simulink model "test_hysteresis_sim"  (R2024a)
settings: Solver=VariableStepAuto  StartTime=0.0  StopTime=10.0  RelTol=1e-3
settings Model: Creator=pichim  LastModifiedBy=pichim

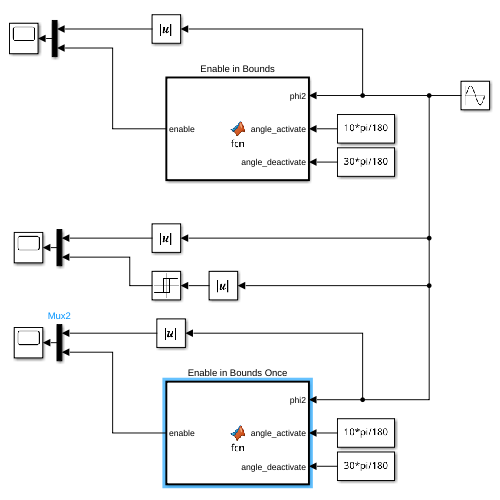
[thumbnail: Simulink's stored preview of the top-level diagram]
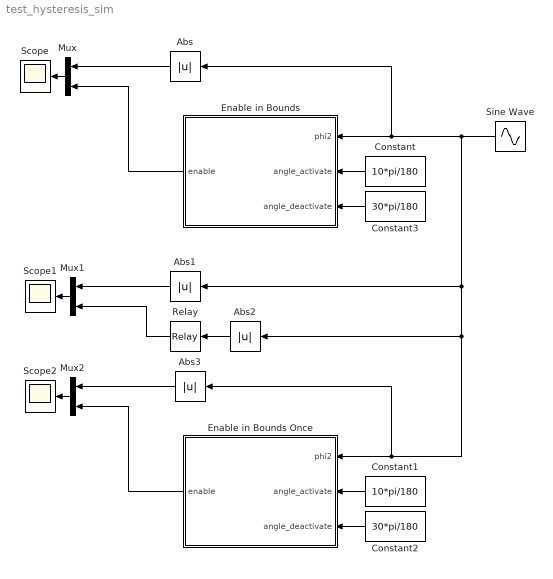
== system test_hysteresis_sim ==
  Abs{,1..3} (4 alike) : Abs  SaturateOnIntegerOverflow=off
  Constant : Constant  Value=10*pi/180
  Constant1 : Constant  Value=10*pi/180
  Constant2 : Constant  Value=30*pi/180
  Constant3 : Constant  Value=30*pi/180
  Enable in Bounds : MATLAB Function  TreatAsAtomicUnit=on
  Enable in Bounds Once : MATLAB Function  TreatAsAtomicUnit=on
  Mux : Mux  Inputs=2
  Mux1 : Mux  Inputs=2
  Mux2 : Mux  Inputs=2
  Relay : Relay  OnSwitchValue=30*pi/180  OffSwitchValue=10*pi/180  OnOutputValue=0  OffOutputValue=1
  Scope : Scope
  Scope1 : Scope
  Scope2 : Scope
  Sine Wave : Sin  SampleTime=0
  wires:
  Constant3/1 -> Enable in Bounds/3(angle_deactivate)
  Constant/1 -> Enable in Bounds/2(angle_activate)
  Mux/1 -> Scope/1
  Enable in Bounds/1(enable) -> Mux/2
  Abs/1 -> Mux/1
  Abs1/1 -> Mux1/1
  Relay/1 -> Mux1/2
  Mux1/1 -> Scope1/1
  Abs2/1 -> Relay/1
  Abs3/1 -> Mux2/1
  Enable in Bounds Once/1(enable) -> Mux2/2
  Mux2/1 -> Scope2/1
  Sine Wave/1 -> Enable in Bounds Once/1(phi2), Abs3/1, Abs2/1, Abs1/1, Abs/1, Enable in Bounds/1(phi2)
  Constant1/1 -> Enable in Bounds Once/2(angle_activate)
  Constant2/1 -> Enable in Bounds Once/3(angle_deactivate)

== matlab function test_hysteresis_sim/Enable in Bounds Once ==
  settings: updateMethod=DISCRETE  sampleTime=Ts
  data: phi2 input; angle_activate input; enable output; angle_deactivate input
function enable = fcn(phi2, angle_activate, angle_deactivate)
% FCN implements a one-shot hysteresis switch:
%  - Activates when   |phi2| < angle_activate   (only if never activated before)
%  - Deactivates when |phi2| > angle_deactivate (after activation)
%  - Cannot be activated again once deactivated
%
% Inputs:
%   phi2              current angle in radians
%   angle_activate    activation threshold (inner) in radians
%   angle_deactivate  deactivation threshold (outer) in radians
%
% Outputs:
%   enable = 1 when active, 0 when inactive (locked after first deactivate)

    persistent active_state has_been_enabled_once
    if isempty(active_state)
        active_state = false;
        has_been_enabled_once = false;
    end

    if ~has_been_enabled_once
        if ~active_state && abs(phi2) < angle_activate
            active_state = true;
        elseif active_state && abs(phi2) > angle_deactivate
            active_state = false;
            has_been_enabled_once = true; % lock out further activations
        end
    end

    enable = double(active_state);
end

== matlab function test_hysteresis_sim/Enable in Bounds ==
  settings: updateMethod=DISCRETE  sampleTime=Ts
  data: phi2 input; angle_activate input; enable output; angle_deactivate input
function enable = fcn(phi2, angle_activate, angle_deactivate)
% FCN implements a hysteresis switch:
%  - Activates when   |phi2| < angle_activate
%  - Deactivates when |phi2| > angle_deactivate
%
% Inputs:
%   phi2              current angle in radians
%   angle_activate    activation threshold (inner) in radians
%   angle_deactivate  deactivation threshold (outer) in radians
%
% Outputs:
%   enable = 1 when active, 0 when inactive

    persistent active_state
    if isempty(active_state)
        active_state = false;
    end

    if ~active_state && abs(phi2) < angle_activate
        active_state = true;
    elseif active_state && abs(phi2) > angle_deactivate
        active_state = false;
    end

    if active_state
        enable = 1;
    else
        enable = 0;
    end
end
